simulink model "obsluga_pwm"  (Simulink 8.4)
settings: Solver=ode45  StartTime=0.0  StopTime=10.0  RelTol=1e-3
settings Model: Creator=Michal  LastModifiedBy=Michal
settings DataIOCC: SignalLoggingSaveFormat=Dataset
settings OptimizationCC: ExpressionDepthLimit=128
settings DebuggingCC: UnderspecifiedInitializationDetection=Simplified  MergeDetectMultiDrivingBlocksExec=error  FcnCallInpInsideContextMsg=EnableAllAsError  StateNameClashWarn=none
settings GRTTargetCC: CombineOutputUpdateFcns=on  GRTInterface=off
settings ConfigComp: Description=PLC Coder Custom Configuration Component  PLC_TargetIDE=pcworx60  PLC_GenerateReport=off

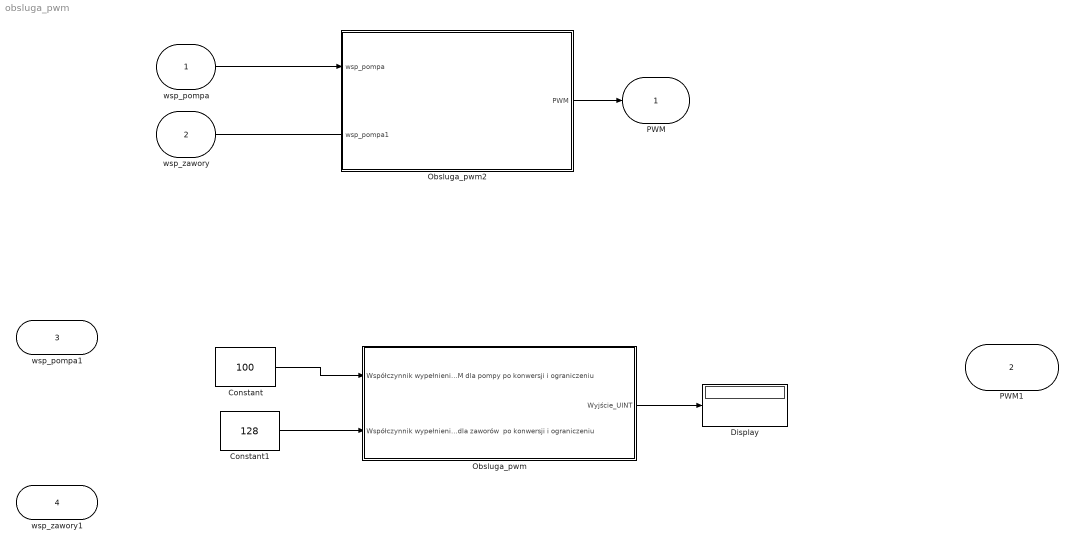
== system obsluga_pwm ==
  wsp_pompa : Inport
  wsp_zawory : Inport  Port=2
  wsp_pompa1 : Inport  Port=3  OutDataTypeStr=uint32
  wsp_zawory1 : Inport  Port=4  OutDataTypeStr=uint32
  Constant : Constant  Value=100  OutDataTypeStr=uint32
  Constant1 : Constant  Value=128  OutDataTypeStr=uint32
  Display : Display
      settings: Format=hex (Stored Integer)
  Obsluga_pwm : Subsystem  TreatAsAtomicUnit=on
  Obsluga_pwm2 : Subsystem  TreatAsAtomicUnit=on
      settings: MinAlgLoopOccurrences=on
  PWM : Outport
  PWM1 : Outport  Port=2  OutDataTypeStr=uint32
  wires:
  wsp_pompa/1 -> Obsluga_pwm2/1(wsp_pompa)
  wsp_zawory/1 -> ?
  Obsluga_pwm2/1(PWM) -> PWM/1
  Constant1/1 -> Obsluga_pwm/2(Współczynnik wypełnienia sygnału PWM dla zaworów  po konwersji i ograniczeniu)
  Constant/1 -> Obsluga_pwm/1(Współczynnik wypełnienia  sygnału PWM dla pompy po konwersji i ograniczeniu)
  Obsluga_pwm/1(Wyjście_UINT) -> Display/1

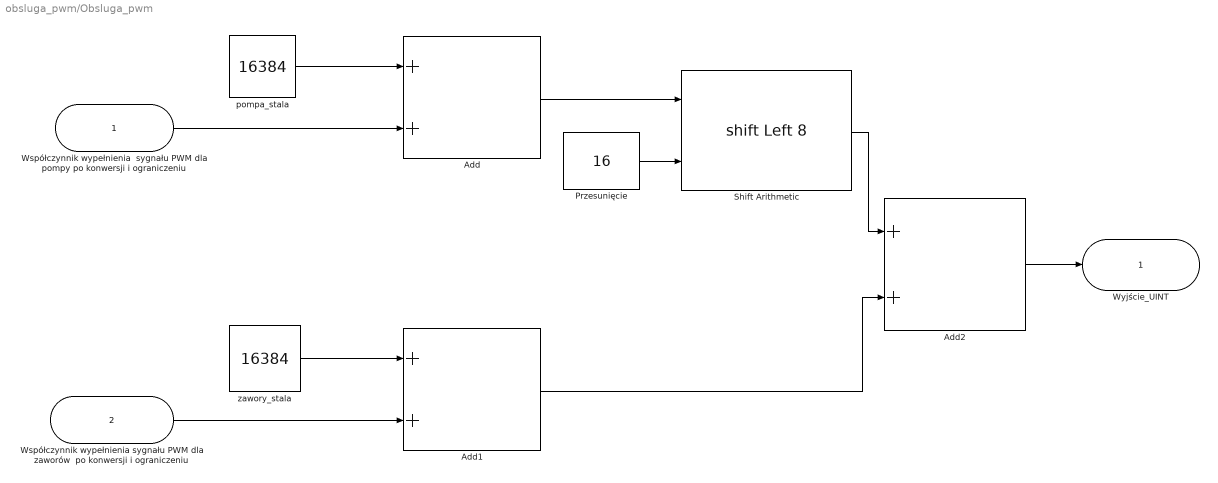
== system obsluga_pwm/Obsluga_pwm ==
  Współczynnik wypełnienia  sygnału PWM dla pompy po konwersji i ograniczeniu : Inport  OutDataTypeStr=uint32
  Współczynnik wypełnienia sygnału PWM dla zaworów  po konwersji i ograniczeniu : Inport  Port=2  OutDataTypeStr=uint32
  Add : Sum
  Add1 : Sum
  Add2 : Sum  AccumDataTypeStr=uint32
  Przesunięcie : Constant  Value=16  OutDataTypeStr=uint8
  Shift Arithmetic : ArithShift  BitShiftNumberSource=Input port  BitShiftNumber=8  BitShiftDirection=Left  DiagnosticForOORShift=Warning
      settings: InputPortMap=u0,p1
  pompa_stala : Constant  Value=16384  OutDataTypeStr=uint32
  zawory_stala : Constant  Value=16384  OutDataTypeStr=uint32
  Wyjście_UINT : Outport  OutDataTypeStr=uint32
  wires:
  Add/1 -> Shift Arithmetic/1
  Add2/1 -> Wyjście_UINT/1
  Przesunięcie/1 -> Shift Arithmetic/2
  zawory_stala/1 -> Add1/1
  Add1/1 -> Add2/2
  pompa_stala/1 -> Add/1
  Współczynnik wypełnienia  sygnału PWM dla pompy po konwersji i ograniczeniu/1 -> Add/2
  Współczynnik wypełnienia sygnału PWM dla zaworów  po konwersji i ograniczeniu/1 -> Add1/2
  Shift Arithmetic/1 -> Add2/1

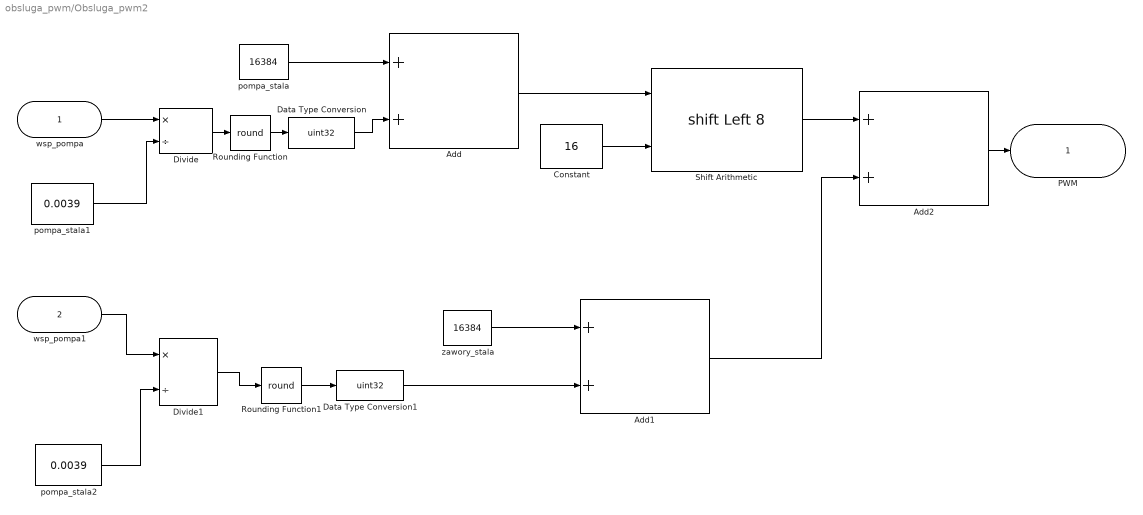
== system obsluga_pwm/Obsluga_pwm2 ==
  wsp_pompa : Inport  OutDataTypeStr=single
  wsp_pompa1 : Inport  Port=2  OutDataTypeStr=single
  Add : Sum
  Add1 : Sum
  Add2 : Sum  AccumDataTypeStr=uint32
  Constant : Constant  Value=16  OutDataTypeStr=uint8
  Data Type Conversion : DataTypeConversion  OutDataTypeStr=uint32
  Data Type Conversion1 : DataTypeConversion  OutDataTypeStr=uint32
  Divide : Product  Inputs=*/
  Divide1 : Product  Inputs=*/
  Rounding Function : Rounding  Operator=round
  Rounding Function1 : Rounding  Operator=round
  Shift Arithmetic : ArithShift  BitShiftNumberSource=Input port  BitShiftNumber=8  BitShiftDirection=Left  DiagnosticForOORShift=Warning
      settings: InputPortMap=u0,p1
  pompa_stala : Constant  Value=16384  OutDataTypeStr=uint32
  pompa_stala1 : Constant  Value=0.0039  OutDataTypeStr=single
  pompa_stala2 : Constant  Value=0.0039  OutDataTypeStr=single
  zawory_stala : Constant  Value=16384  OutDataTypeStr=uint32
  PWM : Outport  OutDataTypeStr=uint32
  wires:
  pompa_stala/1 -> Add/1
  Add/1 -> Shift Arithmetic/1
  Add2/1 -> PWM/1
  Constant/1 -> Shift Arithmetic/2
  zawory_stala/1 -> Add1/1
  Add1/1 -> Add2/2
  Shift Arithmetic/1 -> Add2/1
  wsp_pompa/1 -> Divide/1
  pompa_stala1/1 -> Divide/2
  Divide/1 -> Rounding Function/1
  Rounding Function/1 -> Data Type Conversion/1
  Data Type Conversion/1 -> Add/2
  pompa_stala2/1 -> Divide1/2
  Rounding Function1/1 -> Data Type Conversion1/1
  Data Type Conversion1/1 -> Add1/2
  Divide1/1 -> Rounding Function1/1
  wsp_pompa1/1 -> Divide1/1
